simulink model "Three_Phase_RL"  (R2021b)
settings: Solver=VariableStepAuto  StartTime=0.0  StopTime=2  RelTol=1e-3
undefined symbols (not defined in the file): a
libraries: spsDetailedThyristorLib x6, spsCurrentMeasurementLib x1, spsVoltageMeasurementLib x1, spsSeriesRLCBranchLib x1, spsThreePhaseVIMeasurementLib x1, spsThreePhaseSourceLib x1, spspowerguiLib x1
settings Model: Creator=2003s  LastModifiedBy=viraj

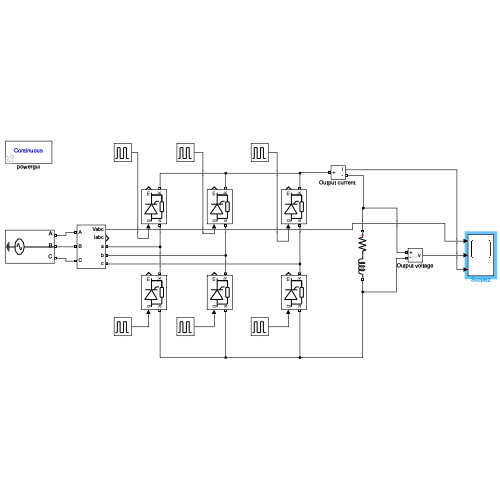
[thumbnail: Simulink's stored preview of the top-level diagram]
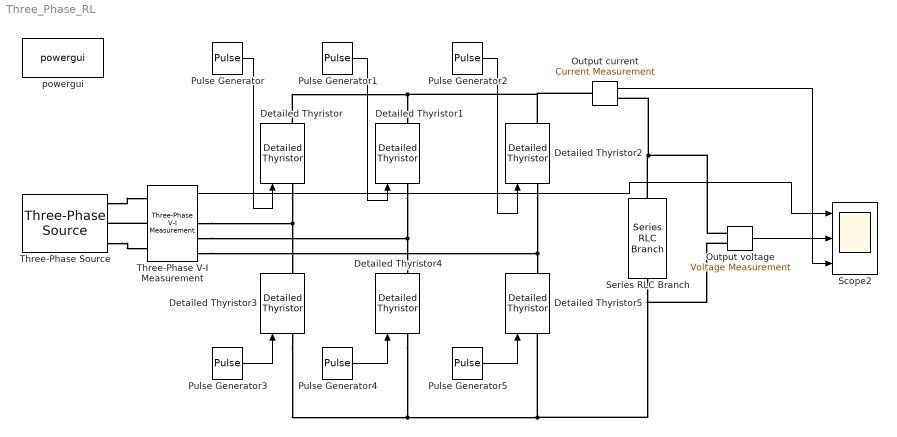
== system Three_Phase_RL ==
  Detailed Thyristor{,1..5} (6 alike) : spsDetailedThyristorLib/Detailed Thyristor  Ron=0.001  Lon=1e-3  Vf=0.8  IL=0.1  Tq=100e-6  IC=0  Rs=500  Cs=250e-9  Measurements=on
      settings: SourceProductBaseCode=PS
  "Output current " : spsCurrentMeasurementLib/Current Measurement  PhasorSimulation=off  OutputType=Complex  PSBequivalent=0
  Output voltage : spsVoltageMeasurementLib/Voltage Measurement  PhasorSimulation=off  OutputType=Complex  PSBequivalent=0
  Pulse Generator : DiscretePulseGenerator  PulseType=Time based  Amplitude=5  Period=0.02  PulseWidth=10  PhaseDelay=a*(0.02/360)
  Pulse Generator1 : DiscretePulseGenerator  PulseType=Time based  Amplitude=5  Period=0.02  PulseWidth=10  PhaseDelay=0.02*((a+120)/360)
  Pulse Generator2 : DiscretePulseGenerator  PulseType=Time based  Amplitude=5  Period=0.02  PulseWidth=10  PhaseDelay=0.02*((a+240)/360)
  Pulse Generator3 : DiscretePulseGenerator  PulseType=Time based  Amplitude=5  Period=0.02  PulseWidth=10  PhaseDelay=0.02*((a+180)/360)
  Pulse Generator4 : DiscretePulseGenerator  PulseType=Time based  Amplitude=5  Period=0.02  PulseWidth=10  PhaseDelay=0.02*((a+300)/360)
  Pulse Generator5 : DiscretePulseGenerator  PulseType=Time based  Amplitude=5  Period=0.02  PulseWidth=10  PhaseDelay=0.02*((a+60)/360)
  Scope2 : Scope  NumInputPorts=3
  Series RLC Branch : spsSeriesRLCBranchLib/Series RLC Branch  LConnTagsString=__new0  RConnTagsString=__new0  BranchType=RL  Resistance=10  Inductance=1e-3  SetiL0=off  InitialCurrent=0  Capacitance=1e-6  Setx0=off  InitialVoltage=0  Measurements=None
  Three-Phase V-I Measurement : spsThreePhaseVIMeasurementLib/Three-Phase V-I Measurement  VoltageMeasurement=phase-to-ground  SetLabelV=off  LabelV=Vabc  Vpu=off  VpuLL=off  CurrentMeasurement=yes  SetLabelI=off  LabelI=Iabc  Ipu=off  Pbase=100e6  Vbase=500e3  OutputType=Complex  PhasorSimulation=off  PSBequivalent=0
  Three-Phase Source : spsThreePhaseSourceLib/Three-Phase Source  InternalConnection=Yg  VoltagePhases=off  Voltage=230  PhaseAngle=0  Voltage_phases=[25e3 25e3 25e3]/sqrt(3)  PhaseAngles_phases=[0 -120 +120]  Frequency=50  NonIdealSource=off  SpecifyImpedance=off  Resistance=0.8929  Inductance=16.58e-3  ShortCircuitLevel=100e6  BaseVoltage=25e3  XRratio=7  BusType=swing  Pref=10e3  Qref=0  Prefabc=[10e3, 10e3, 10e3]  Qrefabc=[0, 0, 0]  Qmin=-inf  Qmax=inf
  powergui : spspowerguiLib/powergui  Priority=1  SimulationMode=Continuous  SampleTime=50e-6  frequency=60  Iterations=50  frequencyindice=50  Pbase=100e6  ErrMax=1e-4  UnitsV=kV  UnitsW=MW  buscounter=0  FunctionMessages=off  echomessages=off  EnableUseOfTLC=off  CurrentSourceSwitches=off  DisableSnubberDevices=off  DisableRonSwitches=off  DisableVfSwitches=off  DisplayEquations=off  AutomaticDiscreteSolvers=off  SolverType=Tustin/Backward Euler (TBE)  Interpol=off  ExternalGateDelay=off  methode=off  Ts=100  x0status=blocks  SPID=on  SwTol=0  HookPort=off  NonlinearTolerance=1e-4  nMaxIteration=100  ContinueOnMaxIteration=off  RestoreLinks=warning  ResistiveCurrentMeasurement=off  Frange=[0:2:500]  Ylog=off  Xlog=on  ShowGrid=off  save=off  variable=ZData  structure=0  ZoomFFT=off  StartTime=0.0  cycles=1  DisplayStyle=1  fundamental=60  FreqAxis=off  MaxFrequency=1000  frequencyindicesteady=1  RmsSteady=1  display=off
  wires:
  Pulse Generator/1 -> Detailed Thyristor/1
  Pulse Generator1/1 -> Detailed Thyristor1/1
  Pulse Generator2/1 -> Detailed Thyristor2/1
  Pulse Generator3/1 -> Detailed Thyristor3/1
  Pulse Generator4/1 -> Detailed Thyristor4/1
  Pulse Generator5/1 -> Detailed Thyristor5/1
  Output voltage/1 -> Scope2/2
  "Output current "/1 -> Scope2/3
  Three-Phase V-I Measurement/1 -> Scope2/1
  connections:
  Detailed Thyristor/RConn1 -- "Output current "/LConn1 -- Detailed Thyristor2/RConn1 -- Detailed Thyristor1/RConn1
  Detailed Thyristor4/LConn1 -- Output voltage/LConn2 -- Series RLC Branch/RConn1 -- Detailed Thyristor5/LConn1 -- Detailed Thyristor3/LConn1
  Detailed Thyristor1/LConn1 -- Three-Phase V-I Measurement/RConn2 -- Detailed Thyristor4/RConn1
  Output voltage/LConn1 -- "Output current "/RConn1 -- Series RLC Branch/LConn1
  Detailed Thyristor/LConn1 -- Three-Phase V-I Measurement/RConn1 -- Detailed Thyristor3/RConn1
  Detailed Thyristor2/LConn1 -- Three-Phase V-I Measurement/RConn3 -- Detailed Thyristor5/RConn1
  Three-Phase Source/RConn1 -- Three-Phase V-I Measurement/LConn1
  Three-Phase V-I Measurement/LConn2 -- Three-Phase Source/RConn2
  Three-Phase Source/RConn3 -- Three-Phase V-I Measurement/LConn3
